simulink library "user_interface"  (R2023b)
settings: Solver=VariableStepAuto  StartTime=0.0  StopTime=10.0  RelTol=1e-3
libraries: input_system x1, seg_display x1
settings Model: Creator=mueller.chris-it22  LastModifiedBy=kilia

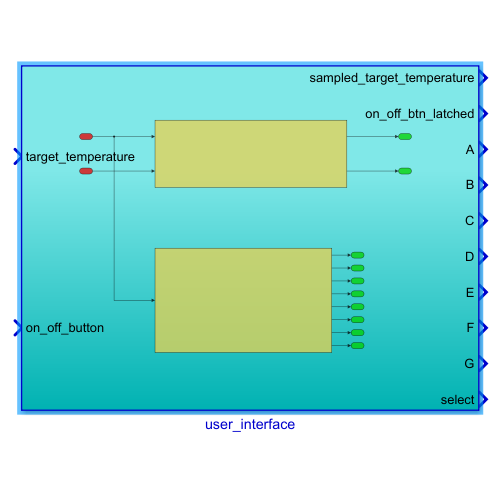
[thumbnail: Simulink's stored preview of the top-level diagram]
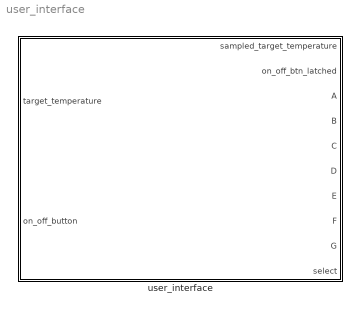
== system user_interface ==
  user_interface : Subsystem

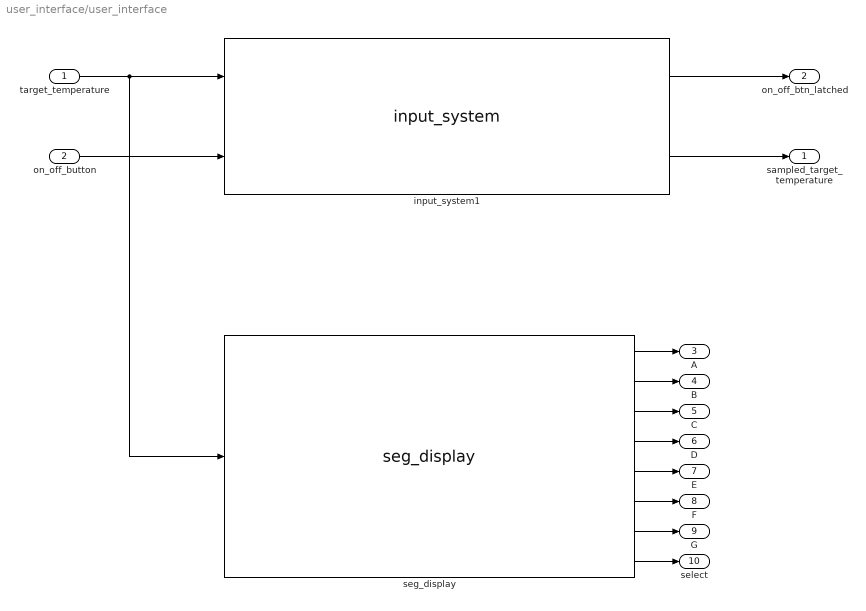
== system user_interface/user_interface ==
  target_temperature : Inport  OutDataTypeStr=uint16
  on_off_button : Inport  Port=2
  input_system1 : input_system/input_system  SystemSampleTime=-1  VariantActivationTime=update diagram  AllowFlexibleInterface=on  Latency=0  AutoFrameSizeCalculation=off
  seg_display : seg_display/seg_display  SystemSampleTime=-1  VariantActivationTime=update diagram  AllowFlexibleInterface=on  Latency=0  AutoFrameSizeCalculation=off
  sampled_target_temperature : Outport
  on_off_btn_latched : Outport  Port=2
  A : Outport  Port=3
  B : Outport  Port=4
  C : Outport  Port=5
  D : Outport  Port=6
  E : Outport  Port=7
  F : Outport  Port=8
  G : Outport  Port=9
  select : Outport  Port=10
  wires:
  input_system1/1 -> on_off_btn_latched/1
  on_off_button/1 -> input_system1/2
  input_system1/2 -> sampled_target_temperature/1
  target_temperature/1 -> seg_display/1, input_system1/1
  seg_display/1 -> A/1
  seg_display/2 -> B/1
  seg_display/3 -> C/1
  seg_display/4 -> D/1
  seg_display/5 -> E/1
  seg_display/6 -> F/1
  seg_display/7 -> G/1
  seg_display/8 -> select/1
